simulink model "FieldOrientedController_RCP"  (R2020b)
settings: configuration reference "SLRT" (kept outside this file)
undefined symbols (not defined in the file): commandTypeEnum, encoder, IO397, pwm, sampleTime
libraries: speedgoatlib_fpga_dio x2, speedgoatlib_fpga_analog_io x2, speedgoatlib_fpga_pwm x2, speedgoatlib_fpga_quadrature x2, speedgoatlib_fpga x2, SignalEditorBlockLib x1
settings Model: DataDictionary=focRCP_Data.sldd  EnableAccessToBaseWorkspace=off  SimulationMode=external  Creator=promero  LastModifiedBy=manuel.fedou
settings ConfigSetRef: SourceName=SLRT

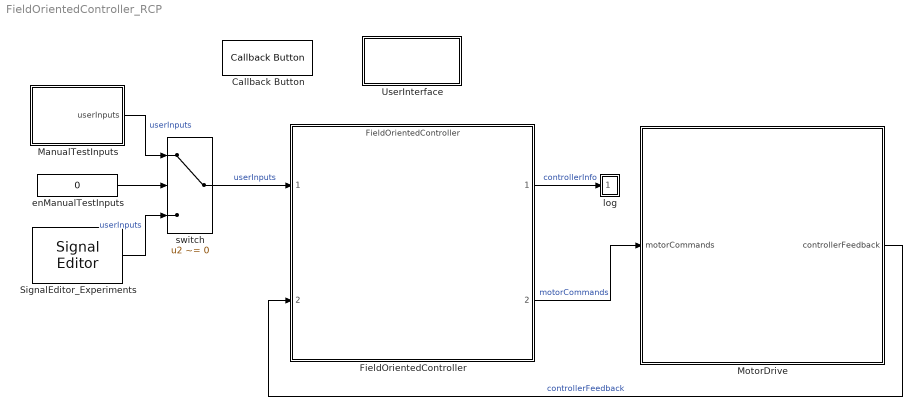
== system FieldOrientedController_RCP ==
  Callback Button : CallbackButton  ButtonText=Switch Electric Motor Control Kit
      settings: ClickFcn=|
      | SelectMotorKit
      | set_param(gcs,'SimulationCommand','Update')
  FieldOrientedController : ModelReference  ModelNameDialog=FieldOrientedController  SimulationMode=Normal  ModelReferenceVersion=1.564
      mask Display: image('focVelocityEncoderHwSwCMask.png');
  ManualTestInputs : Subsystem  Description=""  VariantControl=TestInputChoice == 2
      settings: RTWSystemCode=Nonreusable function
  MotorDrive : Subsystem  Variant=on  VariantControl=demoMode == 2
      mask Display:
      | dd=Simulink.data.dictionary.open('focDemo_Data.sldd');
      | switch getValue(getEntry(dd.getSection('Design Data'),'kitType'))
      |     case 2
      |     image('OldKit.jpg');
      |     case 1
      |     image('NewKit.png');
      |     case 3
      |     image('OldKit.jpg');
      | end
      | clear dd
  SignalEditor_Experiments : SignalEditorBlockLib/Signal Editor  FileName=PMSM_Experiments.mat  ActiveScenario=ClosedLoop_CoastdownTest  ActiveSignal=userInputs  IsBus=on  OutputBusObjectStr=Bus: userInputs  SampleTime=sampleTime.VelocityControl  Interpolate=off  ZeroCross=off  OutputAfterFinalValue=Holding final value  Unit=inherit  PreserveSignalName=on
  UserInterface : Subsystem
  enManualTestInputs : Constant  Value=0  OutDataTypeStr=boolean
  log : Subsystem
  switch : Switch  Criteria=u2 ~= 0
  wires:
  FieldOrientedController/2 -> MotorDrive/1("motorCommands  ")  "motorCommands"
  MotorDrive/1(" controllerFeedback") -> FieldOrientedController/2  "controllerFeedback"
  SignalEditor_Experiments/1 -> switch/3  "userInputs"
  ManualTestInputs/1(userInputs) -> switch/1  "userInputs"
  switch/1 -> FieldOrientedController/1  "userInputs"
  enManualTestInputs/1 -> switch/2
  FieldOrientedController/1 -> log/1(In)  "controllerInfo"

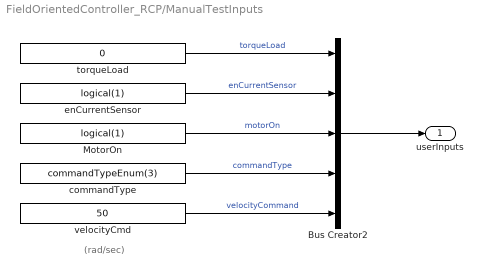
== system FieldOrientedController_RCP/ManualTestInputs ==
  note: (rad/sec)
  Bus Creator2 : BusCreator  Inputs=5  OutDataTypeStr=Bus: userInputs  NonVirtualBus=on
      settings: InheritFromInputs=off
  MotorOn : Constant  Value=logical(1)  OutDataTypeStr=boolean  SampleTime=sampleTime.VelocityControl
  commandType : Constant  Value=commandTypeEnum(3)  SampleTime=sampleTime.VelocityControl
  enCurrentSensor : Constant  Value=logical(1)  OutDataTypeStr=boolean  SampleTime=sampleTime.VelocityControl
  torqueLoad : Constant  Value=0  OutDataTypeStr=double  SampleTime=sampleTime.VelocityControl
  velocityCmd : Constant  Value=50  OutDataTypeStr=single  SampleTime=sampleTime.VelocityControl
  userInputs : Outport  VectorParamsAs1DForOutWhenUnconnected=off
  wires:
  MotorOn/1 -> Bus Creator2/3  "motorOn"
  commandType/1 -> Bus Creator2/4  "commandType"
  torqueLoad/1 -> Bus Creator2/1  "torqueLoad"
  enCurrentSensor/1 -> Bus Creator2/2  "enCurrentSensor"
  Bus Creator2/1 -> userInputs/1
  velocityCmd/1 -> Bus Creator2/5  "velocityCommand"

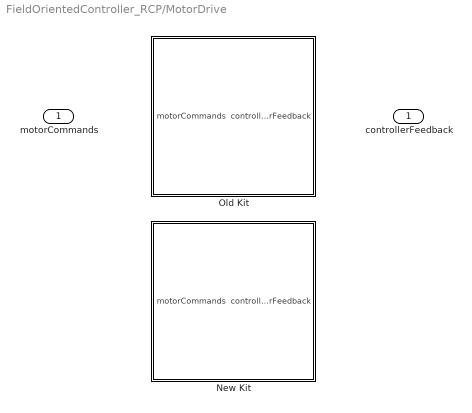
== system FieldOrientedController_RCP/MotorDrive ==
  "motorCommands  " : Inport
  New Kit : Subsystem  VariantControl=kitType == 1
      mask Display: image('NewKit.png'); % Use "Edit Image" on toolstrip to change.
  Old Kit : Subsystem  VariantControl=kitType == 2
      mask Display: image('OldKit.jpg'); % Use "Edit Image" on toolstrip to change.
  " controllerFeedback" : Outport  OutDataTypeStr=Bus: controllerFeedback  VectorParamsAs1DForOutWhenUnconnected=off

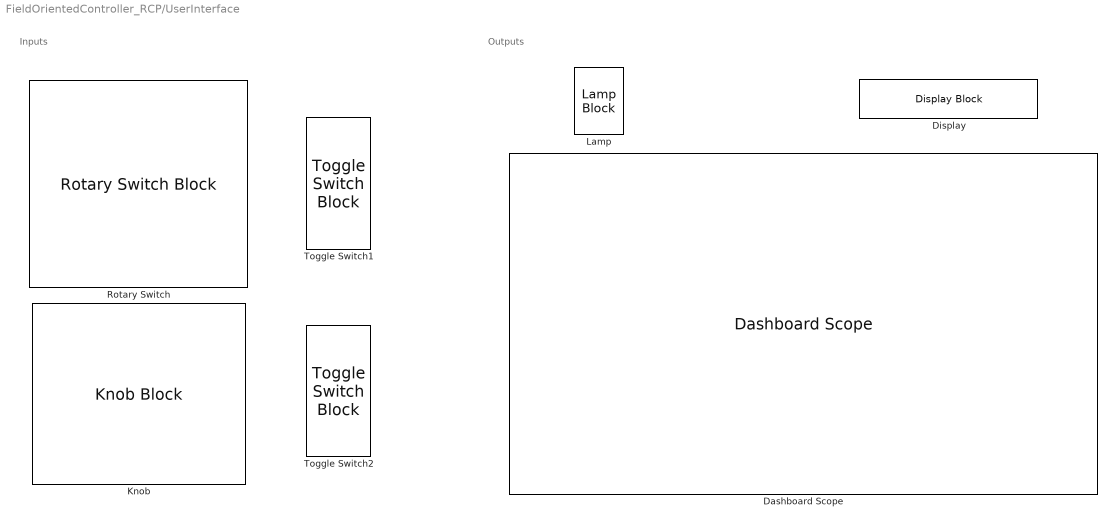
== system FieldOrientedController_RCP/UserInterface ==
  note: Inputs
  note: Outputs
  Dashboard Scope : DashboardScope  TimeSpan=10  Ymin=-250  Ymax=250  ScaleAtStop=off
  Display : DisplayBlock  LabelPosition=Hide  Format=short  Transparency=1
  Knob : KnobBlock  ScaleMin=-250  ScaleMax=250  TickInterval=50
  Lamp : LampBlock
  Rotary Switch : RotarySwitchBlock  UseEnumeratedDataType=on  EnumeratedDataType=commandTypeEnum
  Toggle Switch1 : ToggleSwitchBlock
      settings: Values={{'Off', 'On'}, [0 1]}
  Toggle Switch2 : ToggleSwitchBlock
      settings: Values={{'Off', 'On'}, [0 1]}

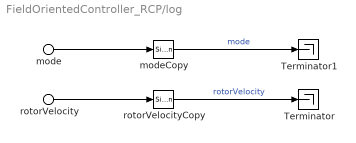
== system FieldOrientedController_RCP/log ==
  mode : Inport  PortName=In  Element=mode
  rotorVelocity : Inport  PortName=In  Element=rotorVelocity
  Terminator : Terminator
  Terminator1 : Terminator
  modeCopy : SignalConversion  OverrideOpt=on
  rotorVelocityCopy : SignalConversion  OverrideOpt=on
  wires:
  rotorVelocity/1 -> rotorVelocityCopy/1
  mode/1 -> modeCopy/1
  rotorVelocityCopy/1 -> Terminator/1  "rotorVelocity"
  modeCopy/1 -> Terminator1/1  "mode"

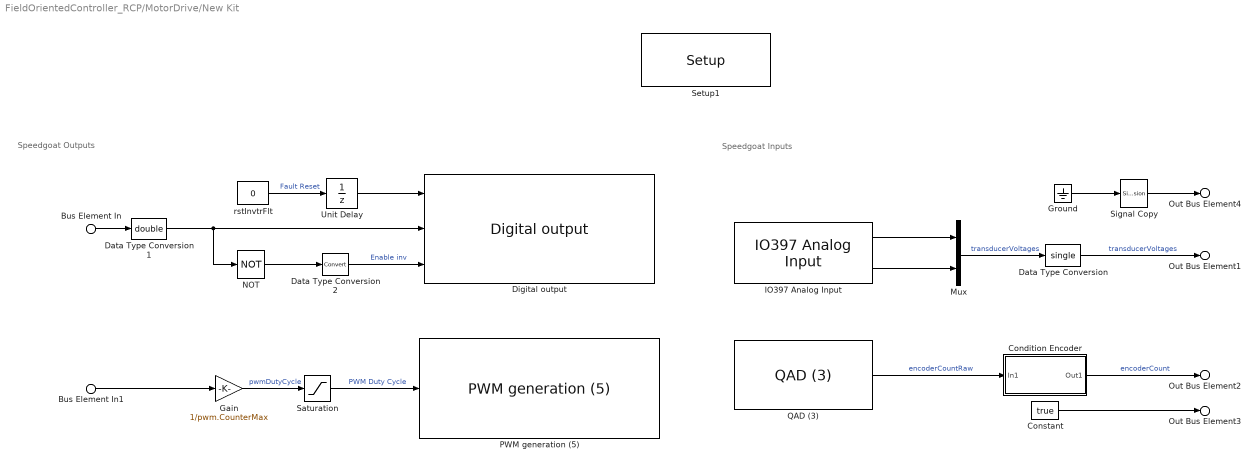
== system FieldOrientedController_RCP/MotorDrive/New Kit ==
  note: Speedgoat Outputs
  note: Speedgoat Inputs
  Bus Element In : Inport  PortName=motorCommands  Element=enInverter
  Bus Element In1 : Inport  PortName=motorCommands  Element=pwmCompare
  Condition Encoder : Subsystem  mask(Speedgoat Encoder Counter){cntsPerRevolution=encoder.CountPerRevolution, positiveDirection=encoder.ALeadsB}
      mask prompts: cntsPerRevolution "Counts per revolution"; positiveDirection "A leads B?"
      mask help: Configures the direction and positive range of the counter value returned by the Speedgoat IO313 QAD Read block.
      mask init:
      | if positiveDirection == 1
      |     strPositiveDirection = 'A Leads B';
      | else
      |     strPositiveDirection = 'B Leads A';
      | end
      mask Display: fprintf(['Encoder\nPositive Direction:\n' strPositiveDirection]);
  Constant : Constant  Value=true  SampleTime=sampleTime.CurrentControl
  Data Type Conversion : DataTypeConversion  OutDataTypeStr=single
  Data Type Conversion1 : DataTypeConversion  OutDataTypeStr=double
  Data Type Conversion2 : DataTypeConversion
  Digital output : speedgoatlib_fpga_dio/Digital output  id=1  chan=[1 4 5]  init=[1 0 0]  reset=[1 1 1]  vectorizeInput=off  ts=-1  pciSlot=-1  board=IO397-50k
      settings: SourceProductName=Simulink Real-Time: Speedgoat I/O Driver Library
  Gain : Gain  Gain=1/pwm.CounterMax  OutDataTypeStr=double
      settings: AttributesFormatString=|
      | --------------------------------
      | Gain = %<Gain>
  Ground : Ground
  IO397 Analog Input : speedgoatlib_fpga_analog_io/IO397 Analog Input  id=1  chan=[1:2]  range=+-5.12 V  trigger=Target  ts=sampleTime.CurrentControl  pciSlot=-1  board=IO397-50k
      settings: SourceProductName=Simulink Real-Time: Speedgoat I/O Driver Library
  Mux : Mux  Inputs=2
  NOT : Logic  Operator=NOT  IconShape=distinctive  AllPortsSameDT=off  OutDataTypeStr=boolean
  PWM generation (5) : speedgoatlib_fpga_pwm/PWM generation (5)  id=1  chan=[1 2 3]  board=IO397-50k  ts=-1  pciSlot=-1  delay=0  symmetric=Symmetric - PWM generation is centered around half the period  b_is_complement_of_a=The complement of PWM A output  deadband=[0.0]  period=pwm.Period  frequency=25000  ticks=2999  a_on=[0]  a_off=[0]  pwm_a_dc=[0.5]  b_on=[0]  b_off=[0]  pwm_b_dc=[0]  c_on=[0.0]  c_off=[0.0]  protection=B is forced off when A is on.  enable_latch_half_period=off  pwm_update=At period starts  trigger_duration=[1e-6]  trigger_period_start=on  trigger_half_of_the_period=off  trigger_a_on=off  trigger_a_off=off  trigger_b_on=off  trigger_b_off=off  show_a_input=on  show_b_input=on  show_c_input=off  show_period_input=off  show_force_stop_input=off  idle_a=Low when PWM generation is halted  idle_b=Low when PWM generation is halted  idle_c=Low when PWM generation is halted  cancels_pwm_generation=on  invert_a=off  invert_b=off  invert_c=off
      settings: SourceProductName=Simulink Real-Time: Speedgoat I/O Driver Library
  QAD (3) : speedgoatlib_fpga_quadrature/QAD (3)  id=1  board=IO397-50k  chan=[1]  resetOnStart=on  ts=sampleTime.CurrentControl  pciSlot=-1  operatingMode=Quadrature decoder  indexControlMode=Ignore index  resolution=4x  stepsPerRevolution=encoder.CountPerRevolution  latchMode=Disabled  interpolatePosition=off  invertAB=off  showClearPositionInput=off  showClearIndexFoundInput=off  showPositionOutput=on  showTurnOutput=off  showSpeedOutput=off  showDirectionOutput=off  showIndexFoundOutput=off
      settings: SourceProductName=Simulink Real-Time: Speedgoat I/O Driver Library
  Saturation : Saturate  UpperLimit=1  LowerLimit=0
  Setup1 : speedgoatlib_fpga/Setup/Setup  board=IO397-50k  id=1  device_id=1  frontIO=None  rearIO=None  bitstreamFile=speedgoat_IO397_50k_CI_02009  rev=1.0  timestamp_string=27/11/19 11:18:03  fpgaFreq=75 MHz  fpgaTick=13.3333 ns  ProgSpiFlash=off  ProgBPIFlash=off  pciSlot=-1  PullRPort0=pull-up 3.3V  VioPort0=3.3V  PullRPort1=pull-up 3.3V  VioPort1=3.3V  PullRPort2=pull-up 3.3V  VioPort2=3.3V  PullRPort3=pull-up 3.3V  VioPort3=3.3V  PullRPort4=pull-up 3.3V  VioPort4=3.3V  PullRPort5=pull-up 3.3V  VioPort5=3.3V  PullRPort6=pull-up 3.3V  VioPort6=3.3V  PullRPort15=pull-up 3.3V  PullRPort31=pull-up 3.3V  PullRPort47=pull-up 3.3V  PullRPort63=pull-up 3.3V
      settings: SourceProductName=Simulink Real-Time: Speedgoat I/O Driver Library
  Signal Copy : SignalConversion  OverrideOpt=off
  Unit Delay : UnitDelay  InitialCondition=1  SampleTime=-1  HasFrameUpgradeWarning=on
  rstInvtrFlt : Constant  Value=0
  Out Bus Element4 : Outport  VectorParamsAs1DForOutWhenUnconnected=off  PortName=controllerFeedback  Element=rotorVelocity
  Out Bus Element1 : Outport  VectorParamsAs1DForOutWhenUnconnected=off  PortName=controllerFeedback  Element=transducerVoltage
  Out Bus Element3 : Outport  VectorParamsAs1DForOutWhenUnconnected=off  PortName=controllerFeedback  Element=encoderIndexFound
  Out Bus Element2 : Outport  VectorParamsAs1DForOutWhenUnconnected=off  PortName=controllerFeedback  Element=encoderCount
  wires:
  Constant/1 -> Out Bus Element3/1
  Gain/1 -> Saturation/1  "pwmDutyCycle"
  Saturation/1 -> PWM generation (5)/1  "PWM Duty Cycle"
  Bus Element In1/1 -> Gain/1
  Condition Encoder/1(Out1) -> Out Bus Element2/1  "encoderCount"
  IO397 Analog Input/2 -> Mux/2
  IO397 Analog Input/1 -> Mux/1
  Data Type Conversion2/1 -> Digital output/3  "Enable inv"
  NOT/1 -> Data Type Conversion2/1
  QAD (3)/1 -> Condition Encoder/1(In1)  "encoderCountRaw"
  Bus Element In/1 -> Data Type Conversion1/1
  Mux/1 -> Data Type Conversion/1  "transducerVoltages"
  rstInvtrFlt/1 -> Unit Delay/1  "Fault Reset"
  Unit Delay/1 -> Digital output/1
  Data Type Conversion/1 -> Out Bus Element1/1  "transducerVoltages"
  Data Type Conversion1/1 -> NOT/1, Digital output/2
  Ground/1 -> Signal Copy/1
  Signal Copy/1 -> Out Bus Element4/1

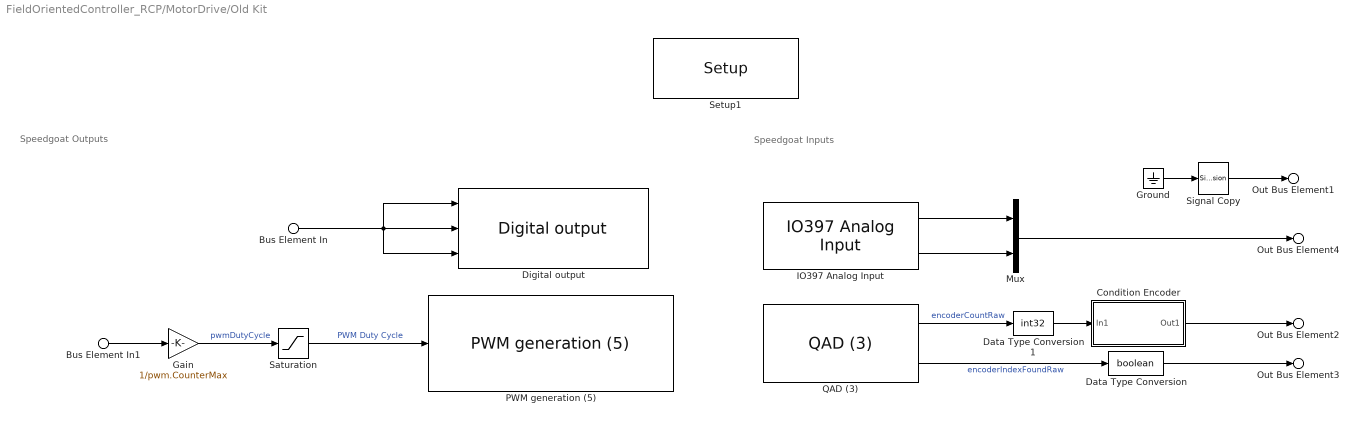
== system FieldOrientedController_RCP/MotorDrive/Old Kit ==
  note: Speedgoat Inputs
  note: Speedgoat Outputs
  Bus Element In : Inport  PortName=motorCommands  Element=enInverter
  Bus Element In1 : Inport  PortName=motorCommands  Element=pwmCompare
  Condition Encoder : Subsystem  mask(Speedgoat Encoder Counter){cntsPerRevolution=encoder.CountPerRevolution, positiveDirection=encoder.ALeadsB}
      mask prompts: cntsPerRevolution "Counts per revolution"; positiveDirection "A leads B?"
      mask help: Configures the direction and positive range of the counter value returned by the Speedgoat IO313 QAD Read block.
      mask init:
      | if positiveDirection == 1
      |     strPositiveDirection = 'A Leads B';
      | else
      |     strPositiveDirection = 'B Leads A';
      | end
      mask Display: fprintf(['Encoder\nPositive Direction:\n' strPositiveDirection]);
  Data Type Conversion : DataTypeConversion  OutDataTypeStr=boolean
  Data Type Conversion1 : DataTypeConversion  OutDataTypeStr=int32
  Digital output : speedgoatlib_fpga_dio/Digital output  id=1  chan=[2:4]  init=0  reset=0  vectorizeInput=off  ts=-1  pciSlot=-1  board=IO397-50k
      settings: SourceProductName=Simulink Real-Time: Speedgoat I/O Driver Library
  Gain : Gain  Gain=1/pwm.CounterMax
      settings: AttributesFormatString=|
      | --------------------------------
      | Gain = %<Gain>
  Ground : Ground
  IO397 Analog Input : speedgoatlib_fpga_analog_io/IO397 Analog Input  id=1  chan=[1:2]  range=+5.12 V  trigger=Target  ts=sampleTime.CurrentControl  pciSlot=-1  board=IO397-50k
      settings: SourceProductName=Simulink Real-Time: Speedgoat I/O Driver Library
  Mux : Mux  Inputs=2
  PWM generation (5) : speedgoatlib_fpga_pwm/PWM generation (5)  id=1  chan=[1 2 3]  board=IO397-50k  ts=-1  pciSlot=-1  delay=0  symmetric=Symmetric - PWM generation is centered around half the period  b_is_complement_of_a=The complement of PWM A output  deadband=[0.0]  period=pwm.Period  frequency=25000  ticks=2999  a_on=[0]  a_off=[0]  pwm_a_dc=[0.5]  b_on=[0]  b_off=[0]  pwm_b_dc=[0]  c_on=[0.0]  c_off=[0.0]  protection=B is forced off when A is on.  enable_latch_half_period=off  pwm_update=At period starts  trigger_duration=[1e-6]  trigger_period_start=on  trigger_half_of_the_period=off  trigger_a_on=off  trigger_a_off=off  trigger_b_on=off  trigger_b_off=off  show_a_input=on  show_b_input=on  show_c_input=off  show_period_input=off  show_force_stop_input=off  idle_a=Low when PWM generation is halted  idle_b=Low when PWM generation is halted  idle_c=Low when PWM generation is halted  cancels_pwm_generation=on  invert_a=off  invert_b=off  invert_c=off
      settings: SourceProductName=Simulink Real-Time: Speedgoat I/O Driver Library
  QAD (3) : speedgoatlib_fpga_quadrature/QAD (3)  id=1  board=IO397-50k  chan=[1]  resetOnStart=on  ts=sampleTime.CurrentControl  pciSlot=-1  operatingMode=Quadrature decoder  indexControlMode=Ignore index  resolution=4x  stepsPerRevolution=encoder.CountPerRevolution  latchMode=Disabled  interpolatePosition=off  invertAB=off  showClearPositionInput=off  showClearIndexFoundInput=off  showPositionOutput=on  showTurnOutput=off  showSpeedOutput=off  showDirectionOutput=off  showIndexFoundOutput=on
      settings: SourceProductName=Simulink Real-Time: Speedgoat I/O Driver Library
  Saturation : Saturate  UpperLimit=1  LowerLimit=0
  Setup1 : speedgoatlib_fpga/Setup/Setup  board=IO397-50k  id=1  device_id=1  frontIO=None  rearIO=None  bitstreamFile=speedgoat_IO397_50k_CI_IO397_PMSM_DEMO  rev=1.0  timestamp_string=23/06/34 18:45:29  fpgaFreq=75 MHz  fpgaTick=13.3333 ns  ProgSpiFlash=off  ProgBPIFlash=off  pciSlot=-1  PullRPort0=pull-up 3.3V  VioPort0=3.3V  PullRPort1=pull-up 3.3V  VioPort1=3.3V  PullRPort2=pull-up 3.3V  VioPort2=3.3V  PullRPort3=pull-up 3.3V  VioPort3=3.3V  PullRPort4=pull-up 3.3V  VioPort4=3.3V  PullRPort5=pull-up 3.3V  VioPort5=3.3V  PullRPort6=pull-up 3.3V  VioPort6=3.3V  PullRPort15=pull-up 3.3V  PullRPort31=pull-up 3.3V  PullRPort47=pull-up 3.3V  PullRPort63=pull-up 3.3V
      settings: SourceProductName=Simulink Real-Time: Speedgoat I/O Driver Library
  Signal Copy : SignalConversion  OverrideOpt=off
  Out Bus Element1 : Outport  VectorParamsAs1DForOutWhenUnconnected=off  PortName=controllerFeedback  Element=rotorVelocity
  Out Bus Element2 : Outport  VectorParamsAs1DForOutWhenUnconnected=off  PortName=controllerFeedback  Element=encoderCount
  Out Bus Element3 : Outport  VectorParamsAs1DForOutWhenUnconnected=off  PortName=controllerFeedback  Element=encoderIndexFound
  Out Bus Element4 : Outport  PortName=controllerFeedback  Element=transducerVoltage
  wires:
  Saturation/1 -> PWM generation (5)/1  "PWM Duty Cycle"
  Bus Element In1/1 -> Gain/1
  Gain/1 -> Saturation/1  "pwmDutyCycle"
  Bus Element In/1 -> Digital output/1, Digital output/3, Digital output/2
  Condition Encoder/1(Out1) -> Out Bus Element2/1
  Mux/1 -> Out Bus Element4/1
  IO397 Analog Input/2 -> Mux/2
  Data Type Conversion1/1 -> Condition Encoder/1(In1)
  QAD (3)/1 -> Data Type Conversion1/1  "encoderCountRaw"
  Data Type Conversion/1 -> Out Bus Element3/1
  QAD (3)/2 -> Data Type Conversion/1  "encoderIndexFoundRaw"
  IO397 Analog Input/1 -> Mux/1
  Ground/1 -> Signal Copy/1
  Signal Copy/1 -> Out Bus Element1/1

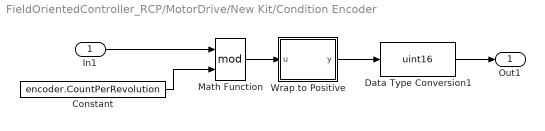
== system FieldOrientedController_RCP/MotorDrive/New Kit/Condition Encoder ==
  In1 : Inport
  Constant : Constant  Value=encoder.CountPerRevolution  OutDataTypeStr=uint32
  Data Type Conversion1 : DataTypeConversion  OutDataTypeStr=uint16
  Math Function : Math  Operator=mod  SignedPower=on  SaturateOnIntegerOverflow=on
  Wrap to Positive : MATLAB Function  TreatAsAtomicUnit=on
  Out1 : Outport  VectorParamsAs1DForOutWhenUnconnected=off
  wires:
  Math Function/1 -> Wrap to Positive/1(u)
  Constant/1 -> Math Function/2
  Wrap to Positive/1(y) -> Data Type Conversion1/1
  In1/1 -> Math Function/1
  Data Type Conversion1/1 -> Out1/1

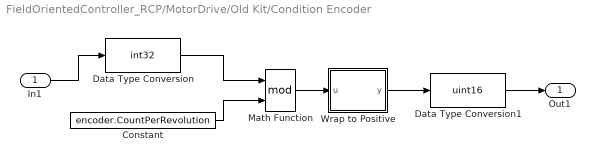
== system FieldOrientedController_RCP/MotorDrive/Old Kit/Condition Encoder ==
  In1 : Inport
  Constant : Constant  Value=encoder.CountPerRevolution  OutDataTypeStr=int32
  Data Type Conversion : DataTypeConversion  OutDataTypeStr=int32
  Data Type Conversion1 : DataTypeConversion  OutDataTypeStr=uint16
  Math Function : Math  Operator=mod  SignedPower=on  SaturateOnIntegerOverflow=on
  Wrap to Positive : MATLAB Function  TreatAsAtomicUnit=on
  Out1 : Outport  VectorParamsAs1DForOutWhenUnconnected=off
  wires:
  Math Function/1 -> Wrap to Positive/1(u)
  Constant/1 -> Math Function/2
  In1/1 -> Data Type Conversion/1
  Wrap to Positive/1(y) -> Data Type Conversion1/1
  Data Type Conversion/1 -> Math Function/1
  Data Type Conversion1/1 -> Out1/1

== matlab function FieldOrientedController_RCP/MotorDrive/Old Kit/Condition Encoder/Wrap to Positive ==
  data: u input; y output; cntsPerRevolution parameter; positiveDirection parameter
function y = fcn(u,cntsPerRevolution,positiveDirection)
% Guarantee the count is between 0 and cntsPerRevolution
% (Speedgoat count can be negative)

% Simplest case
y=u;

% % Max consecutive index pulses that can be missed
% maxIndexPulseMissesToRecoverFrom = 2;
% 
% for index = 1:maxIndexPulseMissesToRecoverFrom
%     if y >= cntsPerRevolution
%         y = y - cntsPerRevolution;
%     elseif y < -cntsPerRevolution
%         y = y + cntsPerRevolution;
%     end
% end
% 
% % Wrap angle to positive value
% if (y<0)
%     y = cntsPerRevolution + y;
% end

% Handle case of swapping encoder A & B signals
if positiveDirection ~= 1
    y = (cntsPerRevolution-1) - y;
end

== matlab function FieldOrientedController_RCP/MotorDrive/New Kit/Condition Encoder/Wrap to Positive ==
  data: u input; y output; cntsPerRevolution parameter; positiveDirection parameter
function y = fcn(u,cntsPerRevolution,positiveDirection)
% Guarantee the count is between 0 and cntsPerRevolution
% (Speedgoat count can be negative)

% Simplest case
y=u;

% % Max consecutive index pulses that can be missed
% maxIndexPulseMissesToRecoverFrom = 2;
% 
% for index = 1:maxIndexPulseMissesToRecoverFrom
%     if y >= cntsPerRevolution
%         y = y - cntsPerRevolution;
%     elseif y < -cntsPerRevolution
%         y = y + cntsPerRevolution;
%     end
% end
% 
% % Wrap angle to positive value
% if (y<0)
%     y = cntsPerRevolution + y;
% end

% Handle case of swapping encoder A & B signals
if positiveDirection ~= 1
    y = (cntsPerRevolution-1) - y;
end
